simulink model "Tipologia4_simulink"  (R2014a)
settings: Solver=ode45  StartTime=0.0  StopTime=100  RelTol=1e-3
libraries: cstblocks x3, simulink x1
settings Model: Creator=giova  LastModifiedBy=giova

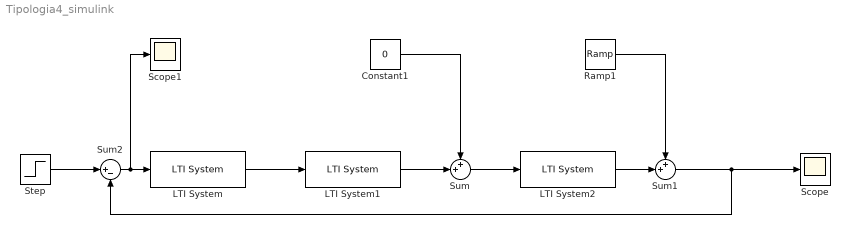
== system Tipologia4_simulink ==
  Constant1 : Constant  Value=0
  LTI System : cstblocks/LTI System  sys=Cz3  IC=[]
  LTI System1 : cstblocks/LTI System  sys=F1  IC=[]
  LTI System2 : cstblocks/LTI System  sys=F2  IC=[]
  Ramp1 : simulink/Sources/Ramp  slope=0  start=0  X0=0
  Scope : Scope
  Scope1 : Scope
  Step : Step  Time=0  SampleTime=0
  Sum : Sum  Inputs=++|
  Sum1 : Sum  Inputs=++|
  Sum2 : Sum  Inputs=|+-
  wires:
  Sum2/1 -> LTI System/1, Scope1/1
  Step/1 -> Sum2/1
  LTI System2/1 -> Sum1/2
  Sum/1 -> LTI System2/1
  LTI System/1 -> LTI System1/1
  LTI System1/1 -> Sum/2
  Sum1/1 -> Sum2/2, Scope/1
  Constant1/1 -> Sum/1
  Ramp1/1 -> Sum1/1
